simulink model "parcial"  (R2022b)
settings: Solver=VariableStepAuto  StartTime=0.0  StopTime=200  RelTol=1e-3
libraries: simulink x1
settings Model: Creator=sophy  LastModifiedBy=sophy

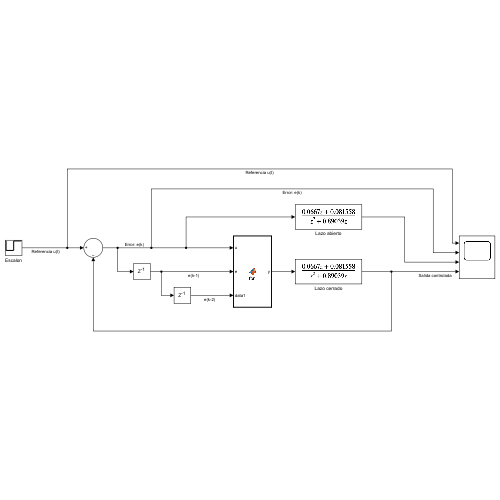
[thumbnail: Simulink's stored preview of the top-level diagram]
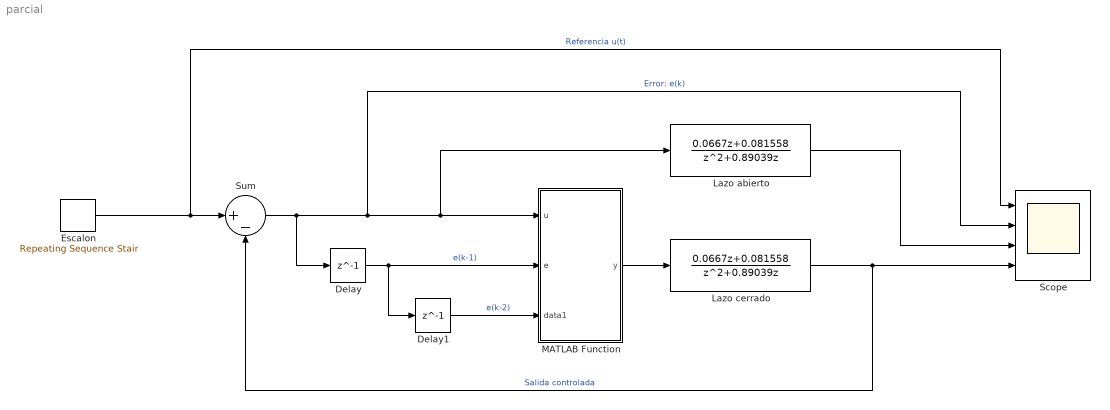
== system parcial ==
  Delay : Delay  DelayLength=1  SampleTime=0.05
  Delay1 : Delay  DelayLength=1  SampleTime=0.05
  Escalon : simulink/Sources/Repeating Sequence Stair  OutValues=[10 20].'  tsamp=100  OutMin=[]  OutMax=[]  OutDataTypeStr=double  OutputDataTypeScalingMode=double  OutDataType=fixdt(0,8)  ConRadixGroup=Best Precision: Vector-wise  OutScaling=2^-12
  Lazo abierto : DiscreteTransferFcn  Numerator=[0.0667 0.081558]  Denominator=[1 0.89039 0]  SampleTime=0.05
  Lazo cerrado : DiscreteTransferFcn  Numerator=[0.0667 0.081558]  Denominator=[1 0.89039 0]  SampleTime=0.05
  MATLAB Function : MATLAB Function  TreatAsAtomicUnit=on
  Scope : Scope  NumInputPorts=4
  Sum : Sum  Inputs=|+-
  wires:
  Sum/1 -> Delay/1, Lazo abierto/1, MATLAB Function/1(u), Scope/2  "Error: e(k)"
  MATLAB Function/1(y) -> Lazo cerrado/1
  Lazo cerrado/1 -> Scope/4, Sum/2  "Salida controlada"
  Escalon/1 -> Sum/1, Scope/1  "Referencia u(t)"
  Delay/1 -> Delay1/1, MATLAB Function/2(e)  "e(k-1)"
  Delay1/1 -> MATLAB Function/3(data1)  "e(k-2)"
  Lazo abierto/1 -> Scope/3

== matlab function parcial/MATLAB Function ==
  data: u input; y output; e input; data1 input
function y = fcn(u, e, data1)

persistent K
if isempty(K)
    K = rand(1);
end

% 
%e = [ek, ek_1, ek_2]/10

u = e*K;

y = u;
